simulink model "baseline_super"  (R2021a)
settings: Solver=FixedStepAuto  StartTime=0.0  StopTime=50  FixedStep=framePeriod_s  RelTol=1e-3
undefined symbols (not defined in the file or in its folder): Aircraft, Earth, framePeriod_s, WGS84
libraries: pid_lib x32, simulink x29, aerolibtransform2 x3, simulink_extras x2, aerolibguid x1
(part 3 of 4)

== system baseline_super/LAND CONTROLLER/Horizontal speed controller/Subsystem ==
  vb_x cmd : Inport
  vb_x : Inport  Port=2
  Constant : Constant  Value=Aircraft.Control.P_v_hor  OutDataTypeStr=single
  Constant1 : Constant  Value=Aircraft.Control.I_v_hor  OutDataTypeStr=single
  Constant2 : Constant  Value=Aircraft.Control.D_v_hor  OutDataTypeStr=single
  Gain : Gain  Gain=-1
  Pitch angle controller : pid_lib/PID Controller  Controller=PID  Form=Parallel  TimeDomain=Discrete-time  UseExternalTs=off  SampleTime=framePeriod_s  IntegratorMethod=Forward Euler  FilterMethod=Forward Euler  ControllerParametersSource=external  P=0.335  I=0.005  D=0  UseFilter=off  N=100  TunerSelectOption=Transfer Function Based (PID Tuner App)  InitialConditionSource=internal  InitialConditionForIntegrator=0  InitialConditionForFilter=0  DifferentiatorICPrevScaledInput=0  ExternalReset=none  TrackingMode=off  Kt=1  LimitOutput=on  SatLimitsSource=internal  UpperSaturationLimit=inf  LowerSaturationLimit=-inf  LinearizeAsGain=off  AntiWindupMode=clamping  Kb=1  POutMin=[]  POutMax=[]  IOutMin=[]  IOutMax=[]  DOutMin=[]  DOutMax=[]  NOutMin=[]  NOutMax=[]  SumOutMin=[]  SumOutMax=[]  SaturationOutMin=[]  SaturationOutMax=[]  PParamMin=[]  PParamMax=[]  IParamMin=[]  IParamMax=[]  DParamMin=[]  DParamMax=[]  NParamMin=[]  NParamMax=[]  KbParamMin=[]  KbParamMax=[]  KtParamMin=[]  KtParamMax=[]  KbOutMin=[]  KbOutMax=[]  KtOutMin=[]  KtOutMax=[]  IntegratorOutMin=[]  IntegratorOutMax=[]  FilterOutMin=[]  FilterOutMax=[]  SumI1OutMin=[]  SumI1OutMax=[]  SumI2OutMin=[]  SumI2OutMax=[]  SumI3OutMin=[]  SumI3OutMax=[]  SumI4OutMin=[]  SumI4OutMax=[]  SumDOutMin=[]  SumDOutMax=[]  DifferentiatorOutMin=[]  DifferentiatorOutMax=[]  FilterDiffOutCoefMin=[]  FilterDiffOutCoefMax=[]  ReciprocalOutMin=[]  ReciprocalOutMax=[]  SumDenOutMin=[]  SumDenOutMax=[]  SumNumOutMin=[]  SumNumOutMax=[]  DivideOutMin=[]  DivideOutMax=[]  UdiffTsProdOutMin=[]  UdiffTsProdOutMax=[]  NTsProdOutMin=[]  NTsProdOutMax=[]  UintegralTsProdOutMin=[]  UintegralTsProdOutMax=[]  UngainTsProdOutMin=[]  UngainTsProdOutMax=[]  IntegratorContinuousStateAttributes=''  IntegratorStateMustResolveToSignalObject=off  IntegratorRTWStateStorageClass=Auto  FilterContinuousStateAttributes=''  FilterStateMustResolveToSignalObject=off  FilterRTWStateStorageClass=Auto  ParallelPVariant=ExternalParameters  IdealPVariant=Disabled  IVariant=ExternalParameters  DVariant=ExternalParameters  IntegratorVariant=Discrete  SatVariant=Enabled  AWVariant=DiscClampingParallel  PCopyVariant=Disabled  TRVariant=Disabled  FdbkBlocksVariant=Forward  IdealPFdbkVariant=Disabled  SatFdbkVariant=Disabled  DerivativeFilterVariant=Differentiator  NVariant=Passthrough  NCopyVariant=Disabled_SignalSpec  FilterICVariant=InternalICsDifferentiator  IntegratorICVariant=InternalICs  ExternalResetVariant=Disabled  TRSumVariant=Passthrough  SumFdbkVariant=Disabled  SumVariant=Sum_PID  TsampFilterVariant=InternalTs  TsampNgainVariant=Passthrough  TsampIntegralVariant=Passthrough  ExternalSaturationOutDataTypeStr=Inherit: Same as second input
  Saturation : Saturate  UpperLimit=Aircraft.Control.pitch_angle_lim  LowerLimit=-Aircraft.Control.pitch_angle_lim  LinearizeAsGain=off
  Sum : Sum  Inputs=|+-
  pitch_cmd_rad : Outport
  wires:
  vb_x/1 -> Sum/2
  Constant1/1 -> Pitch angle controller/3
  Constant2/1 -> Pitch angle controller/4
  Sum/1 -> Pitch angle controller/1
  Constant/1 -> Pitch angle controller/2
  vb_x cmd/1 -> Sum/1
  Saturation/1 -> Gain/1
  Pitch angle controller/1 -> Saturation/1
  Gain/1 -> pitch_cmd_rad/1

== system baseline_super/LAND CONTROLLER/Horizontal speed controller/Subsystem1 ==
  vb_y cmd : Inport
  vb_y : Inport  Port=2
  Constant : Constant  Value=Aircraft.Control.P_v_hor  OutDataTypeStr=single
  Constant1 : Constant  Value=Aircraft.Control.I_v_hor  OutDataTypeStr=single
  Constant2 : Constant  Value=Aircraft.Control.D_v_hor  OutDataTypeStr=single
  Roll angle controller : pid_lib/PID Controller  Controller=PID  Form=Parallel  TimeDomain=Discrete-time  UseExternalTs=off  SampleTime=framePeriod_s  IntegratorMethod=Forward Euler  FilterMethod=Forward Euler  ControllerParametersSource=external  P=0.335  I=0.005  D=0  UseFilter=off  N=100  TunerSelectOption=Transfer Function Based (PID Tuner App)  InitialConditionSource=internal  InitialConditionForIntegrator=0  InitialConditionForFilter=0  DifferentiatorICPrevScaledInput=0  ExternalReset=none  TrackingMode=off  Kt=1  LimitOutput=on  SatLimitsSource=internal  UpperSaturationLimit=inf  LowerSaturationLimit=-inf  LinearizeAsGain=off  AntiWindupMode=clamping  Kb=1  POutMin=[]  POutMax=[]  IOutMin=[]  IOutMax=[]  DOutMin=[]  DOutMax=[]  NOutMin=[]  NOutMax=[]  SumOutMin=[]  SumOutMax=[]  SaturationOutMin=[]  SaturationOutMax=[]  PParamMin=[]  PParamMax=[]  IParamMin=[]  IParamMax=[]  DParamMin=[]  DParamMax=[]  NParamMin=[]  NParamMax=[]  KbParamMin=[]  KbParamMax=[]  KtParamMin=[]  KtParamMax=[]  KbOutMin=[]  KbOutMax=[]  KtOutMin=[]  KtOutMax=[]  IntegratorOutMin=[]  IntegratorOutMax=[]  FilterOutMin=[]  FilterOutMax=[]  SumI1OutMin=[]  SumI1OutMax=[]  SumI2OutMin=[]  SumI2OutMax=[]  SumI3OutMin=[]  SumI3OutMax=[]  SumI4OutMin=[]  SumI4OutMax=[]  SumDOutMin=[]  SumDOutMax=[]  DifferentiatorOutMin=[]  DifferentiatorOutMax=[]  FilterDiffOutCoefMin=[]  FilterDiffOutCoefMax=[]  ReciprocalOutMin=[]  ReciprocalOutMax=[]  SumDenOutMin=[]  SumDenOutMax=[]  SumNumOutMin=[]  SumNumOutMax=[]  DivideOutMin=[]  DivideOutMax=[]  UdiffTsProdOutMin=[]  UdiffTsProdOutMax=[]  NTsProdOutMin=[]  NTsProdOutMax=[]  UintegralTsProdOutMin=[]  UintegralTsProdOutMax=[]  UngainTsProdOutMin=[]  UngainTsProdOutMax=[]  IntegratorContinuousStateAttributes=''  IntegratorStateMustResolveToSignalObject=off  IntegratorRTWStateStorageClass=Auto  FilterContinuousStateAttributes=''  FilterStateMustResolveToSignalObject=off  FilterRTWStateStorageClass=Auto  ParallelPVariant=ExternalParameters  IdealPVariant=Disabled  IVariant=ExternalParameters  DVariant=ExternalParameters  IntegratorVariant=Discrete  SatVariant=Enabled  AWVariant=DiscClampingParallel  PCopyVariant=Disabled  TRVariant=Disabled  FdbkBlocksVariant=Forward  IdealPFdbkVariant=Disabled  SatFdbkVariant=Disabled  DerivativeFilterVariant=Differentiator  NVariant=Passthrough  NCopyVariant=Disabled_SignalSpec  FilterICVariant=InternalICsDifferentiator  IntegratorICVariant=InternalICs  ExternalResetVariant=Disabled  TRSumVariant=Passthrough  SumFdbkVariant=Disabled  SumVariant=Sum_PID  TsampFilterVariant=InternalTs  TsampNgainVariant=Passthrough  TsampIntegralVariant=Passthrough  ExternalSaturationOutDataTypeStr=Inherit: Same as second input
  Saturation : Saturate  UpperLimit=Aircraft.Control.pitch_angle_lim  LowerLimit=-Aircraft.Control.pitch_angle_lim  LinearizeAsGain=off
  Sum : Sum  Inputs=|+-
  roll_cmd_rad : Outport
  wires:
  vb_y/1 -> Sum/2
  Constant1/1 -> Roll angle controller/3
  Constant2/1 -> Roll angle controller/4
  Sum/1 -> Roll angle controller/1
  Constant/1 -> Roll angle controller/2
  vb_y cmd/1 -> Sum/1
  Saturation/1 -> roll_cmd_rad/1
  Roll angle controller/1 -> Saturation/1

== system baseline_super/LAND CONTROLLER/auto_disarm/disarm motor ==
  Enable : EnablePort  StatesWhenEnabling=reset
  Compare To Constant2 : simulink/Logic and Bit Operations/Compare To Constant  relop=>  const=10  OutDataTypeStr=boolean
  Constant : Constant  Value=framePeriod_s
  Sum : Sum  Inputs=|++
  Trigger RTL : Subsystem
  Unit Delay : UnitDelay  SampleTime=-1  HasFrameUpgradeWarning=on
  wires:
  Compare To Constant2/1 -> Trigger RTL/Enable
  Sum/1 -> Compare To Constant2/1, Unit Delay/1
  Unit Delay/1 -> Sum/2
  Constant/1 -> Sum/1

== system baseline_super/POS_HOLD CONTROLLER/Horizontal speed controller/2D rotation from NED_xy to body_xy ==
  <heading_rad> : Inport
  Cos : Trigonometry  Operator=cos  OutputSignalType=real
  Gain : Gain  Gain=-1
  Mux : Mux
  Reshape : Reshape  OutputDimensionality=Customize  OutputDimensions=[2,2]
  Sin : Trigonometry  OutputSignalType=real
  2D_rot : Outport
  wires:
  <heading_rad>/1 -> Sin/1, Cos/1
  Mux/1 -> Reshape/1
  Sin/1 -> Mux/3, Gain/1
  Cos/1 -> Mux/1, Mux/4
  Reshape/1 -> 2D_rot/1
  Gain/1 -> Mux/2

== system baseline_super/POS_HOLD CONTROLLER/Horizontal speed controller/Pitch Controller ==
  pitch_cmd_rad : Inport
  pitch_rad : Inport  Port=2
  D_pitch_angle : Constant  Value=Aircraft.Control.I_pitch_angle  OutDataTypeStr=single
  I_pitch_angle : Constant  Value=Aircraft.Control.D_pitch_angle  OutDataTypeStr=single
  P_pitch_angle : Constant  Value=Aircraft.Control.P_pitch_angle  OutDataTypeStr=single
  Pitch angle controller : pid_lib/PID Controller  Controller=PID  Form=Parallel  TimeDomain=Discrete-time  UseExternalTs=off  SampleTime=framePeriod_s  IntegratorMethod=Forward Euler  FilterMethod=Forward Euler  ControllerParametersSource=external  P=0.335  I=0.005  D=0  UseFilter=off  N=100  TunerSelectOption=Transfer Function Based (PID Tuner App)  InitialConditionSource=internal  InitialConditionForIntegrator=0  InitialConditionForFilter=0  DifferentiatorICPrevScaledInput=0  ExternalReset=none  TrackingMode=off  Kt=1  LimitOutput=on  SatLimitsSource=internal  UpperSaturationLimit=inf  LowerSaturationLimit=-inf  LinearizeAsGain=off  AntiWindupMode=clamping  Kb=1  POutMin=[]  POutMax=[]  IOutMin=[]  IOutMax=[]  DOutMin=[]  DOutMax=[]  NOutMin=[]  NOutMax=[]  SumOutMin=[]  SumOutMax=[]  SaturationOutMin=[]  SaturationOutMax=[]  PParamMin=[]  PParamMax=[]  IParamMin=[]  IParamMax=[]  DParamMin=[]  DParamMax=[]  NParamMin=[]  NParamMax=[]  KbParamMin=[]  KbParamMax=[]  KtParamMin=[]  KtParamMax=[]  KbOutMin=[]  KbOutMax=[]  KtOutMin=[]  KtOutMax=[]  IntegratorOutMin=[]  IntegratorOutMax=[]  FilterOutMin=[]  FilterOutMax=[]  SumI1OutMin=[]  SumI1OutMax=[]  SumI2OutMin=[]  SumI2OutMax=[]  SumI3OutMin=[]  SumI3OutMax=[]  SumI4OutMin=[]  SumI4OutMax=[]  SumDOutMin=[]  SumDOutMax=[]  DifferentiatorOutMin=[]  DifferentiatorOutMax=[]  FilterDiffOutCoefMin=[]  FilterDiffOutCoefMax=[]  ReciprocalOutMin=[]  ReciprocalOutMax=[]  SumDenOutMin=[]  SumDenOutMax=[]  SumNumOutMin=[]  SumNumOutMax=[]  DivideOutMin=[]  DivideOutMax=[]  UdiffTsProdOutMin=[]  UdiffTsProdOutMax=[]  NTsProdOutMin=[]  NTsProdOutMax=[]  UintegralTsProdOutMin=[]  UintegralTsProdOutMax=[]  UngainTsProdOutMin=[]  UngainTsProdOutMax=[]  IntegratorContinuousStateAttributes=''  IntegratorStateMustResolveToSignalObject=off  IntegratorRTWStateStorageClass=Auto  FilterContinuousStateAttributes=''  FilterStateMustResolveToSignalObject=off  FilterRTWStateStorageClass=Auto  ParallelPVariant=ExternalParameters  IdealPVariant=Disabled  IVariant=ExternalParameters  DVariant=ExternalParameters  IntegratorVariant=Discrete  SatVariant=Enabled  AWVariant=DiscClampingParallel  PCopyVariant=Disabled  TRVariant=Disabled  FdbkBlocksVariant=Forward  IdealPFdbkVariant=Disabled  SatFdbkVariant=Disabled  DerivativeFilterVariant=Differentiator  NVariant=Passthrough  NCopyVariant=Disabled_SignalSpec  FilterICVariant=InternalICsDifferentiator  IntegratorICVariant=InternalICs  ExternalResetVariant=Disabled  TRSumVariant=Passthrough  SumFdbkVariant=Disabled  SumVariant=Sum_PID  TsampFilterVariant=InternalTs  TsampNgainVariant=Passthrough  TsampIntegralVariant=Passthrough  ExternalSaturationOutDataTypeStr=Inherit: Same as second input
  Saturation : Saturate  UpperLimit=Aircraft.Control.pitch_rate_max  LowerLimit=-Aircraft.Control.pitch_rate_max
  Sum2 : Sum  Inputs=|+-
  pitch_cc : Outport
  wires:
  Sum2/1 -> Pitch angle controller/1  "pitch error"
  P_pitch_angle/1 -> Pitch angle controller/2
  I_pitch_angle/1 -> Pitch angle controller/3
  pitch_cmd_rad/1 -> Sum2/1  "pitch angle cmd"
  D_pitch_angle/1 -> Pitch angle controller/4
  Pitch angle controller/1 -> Saturation/1
  pitch_rad/1 -> Sum2/2
  Saturation/1 -> pitch_cc/1

== system baseline_super/POS_HOLD CONTROLLER/Horizontal speed controller/Roll Controller ==
  roll_cmd_rad : Inport
  roll_rad : Inport  Port=2
  D_roll_angle : Constant  Value=Aircraft.Control.D_roll_angle  OutDataTypeStr=single
  I_roll_angle : Constant  Value=Aircraft.Control.I_roll_angle  OutDataTypeStr=single
  PID Controller1 : pid_lib/PID Controller  Controller=PID  Form=Parallel  TimeDomain=Discrete-time  UseExternalTs=off  SampleTime=framePeriod_s  IntegratorMethod=Forward Euler  FilterMethod=Forward Euler  ControllerParametersSource=external  P=0.335  I=0.005  D=0  UseFilter=off  N=100  TunerSelectOption=Transfer Function Based (PID Tuner App)  InitialConditionSource=internal  InitialConditionForIntegrator=0  InitialConditionForFilter=0  DifferentiatorICPrevScaledInput=0  ExternalReset=none  TrackingMode=off  Kt=1  LimitOutput=on  SatLimitsSource=internal  UpperSaturationLimit=inf  LowerSaturationLimit=-inf  LinearizeAsGain=off  AntiWindupMode=clamping  Kb=1  POutMin=[]  POutMax=[]  IOutMin=[]  IOutMax=[]  DOutMin=[]  DOutMax=[]  NOutMin=[]  NOutMax=[]  SumOutMin=[]  SumOutMax=[]  SaturationOutMin=[]  SaturationOutMax=[]  PParamMin=[]  PParamMax=[]  IParamMin=[]  IParamMax=[]  DParamMin=[]  DParamMax=[]  NParamMin=[]  NParamMax=[]  KbParamMin=[]  KbParamMax=[]  KtParamMin=[]  KtParamMax=[]  KbOutMin=[]  KbOutMax=[]  KtOutMin=[]  KtOutMax=[]  IntegratorOutMin=[]  IntegratorOutMax=[]  FilterOutMin=[]  FilterOutMax=[]  SumI1OutMin=[]  SumI1OutMax=[]  SumI2OutMin=[]  SumI2OutMax=[]  SumI3OutMin=[]  SumI3OutMax=[]  SumI4OutMin=[]  SumI4OutMax=[]  SumDOutMin=[]  SumDOutMax=[]  DifferentiatorOutMin=[]  DifferentiatorOutMax=[]  FilterDiffOutCoefMin=[]  FilterDiffOutCoefMax=[]  ReciprocalOutMin=[]  ReciprocalOutMax=[]  SumDenOutMin=[]  SumDenOutMax=[]  SumNumOutMin=[]  SumNumOutMax=[]  DivideOutMin=[]  DivideOutMax=[]  UdiffTsProdOutMin=[]  UdiffTsProdOutMax=[]  NTsProdOutMin=[]  NTsProdOutMax=[]  UintegralTsProdOutMin=[]  UintegralTsProdOutMax=[]  UngainTsProdOutMin=[]  UngainTsProdOutMax=[]  IntegratorContinuousStateAttributes=''  IntegratorStateMustResolveToSignalObject=off  IntegratorRTWStateStorageClass=Auto  FilterContinuousStateAttributes=''  FilterStateMustResolveToSignalObject=off  FilterRTWStateStorageClass=Auto  ParallelPVariant=ExternalParameters  IdealPVariant=Disabled  IVariant=ExternalParameters  DVariant=ExternalParameters  IntegratorVariant=Discrete  SatVariant=Enabled  AWVariant=DiscClampingParallel  PCopyVariant=Disabled  TRVariant=Disabled  FdbkBlocksVariant=Forward  IdealPFdbkVariant=Disabled  SatFdbkVariant=Disabled  DerivativeFilterVariant=Differentiator  NVariant=Passthrough  NCopyVariant=Disabled_SignalSpec  FilterICVariant=InternalICsDifferentiator  IntegratorICVariant=InternalICs  ExternalResetVariant=Disabled  TRSumVariant=Passthrough  SumFdbkVariant=Disabled  SumVariant=Sum_PID  TsampFilterVariant=InternalTs  TsampNgainVariant=Passthrough  TsampIntegralVariant=Passthrough  ExternalSaturationOutDataTypeStr=Inherit: Same as second input
  P_roll_angle : Constant  Value=Aircraft.Control.P_roll_angle  OutDataTypeStr=single
  Saturation : Saturate  UpperLimit=Aircraft.Control.roll_rate_max  LowerLimit=-Aircraft.Control.roll_rate_max
  Sum : Sum  Inputs=|+-
  roll_cc : Outport
  wires:
  PID Controller1/1 -> Saturation/1  "Roll_cmd"
  roll_cmd_rad/1 -> Sum/1  "roll_angle_command"
  Sum/1 -> PID Controller1/1  "roll_angle_error"
  P_roll_angle/1 -> PID Controller1/2
  I_roll_angle/1 -> PID Controller1/3
  D_roll_angle/1 -> PID Controller1/4
  roll_rad/1 -> Sum/2
  Saturation/1 -> roll_cc/1

== system baseline_super/POS_HOLD CONTROLLER/Horizontal speed controller/Subsystem ==
  vb_x cmd : Inport
  vb_x : Inport  Port=2
  Constant : Constant  Value=Aircraft.Control.P_v_hor  OutDataTypeStr=single
  Constant1 : Constant  Value=Aircraft.Control.I_v_hor  OutDataTypeStr=single
  Constant2 : Constant  Value=Aircraft.Control.D_v_hor  OutDataTypeStr=single
  Gain : Gain  Gain=-1
  Pitch angle controller : pid_lib/PID Controller  Controller=PID  Form=Parallel  TimeDomain=Discrete-time  UseExternalTs=off  SampleTime=framePeriod_s  IntegratorMethod=Forward Euler  FilterMethod=Forward Euler  ControllerParametersSource=external  P=0.335  I=0.005  D=0  UseFilter=off  N=100  TunerSelectOption=Transfer Function Based (PID Tuner App)  InitialConditionSource=internal  InitialConditionForIntegrator=0  InitialConditionForFilter=0  DifferentiatorICPrevScaledInput=0  ExternalReset=none  TrackingMode=off  Kt=1  LimitOutput=on  SatLimitsSource=internal  UpperSaturationLimit=inf  LowerSaturationLimit=-inf  LinearizeAsGain=off  AntiWindupMode=clamping  Kb=1  POutMin=[]  POutMax=[]  IOutMin=[]  IOutMax=[]  DOutMin=[]  DOutMax=[]  NOutMin=[]  NOutMax=[]  SumOutMin=[]  SumOutMax=[]  SaturationOutMin=[]  SaturationOutMax=[]  PParamMin=[]  PParamMax=[]  IParamMin=[]  IParamMax=[]  DParamMin=[]  DParamMax=[]  NParamMin=[]  NParamMax=[]  KbParamMin=[]  KbParamMax=[]  KtParamMin=[]  KtParamMax=[]  KbOutMin=[]  KbOutMax=[]  KtOutMin=[]  KtOutMax=[]  IntegratorOutMin=[]  IntegratorOutMax=[]  FilterOutMin=[]  FilterOutMax=[]  SumI1OutMin=[]  SumI1OutMax=[]  SumI2OutMin=[]  SumI2OutMax=[]  SumI3OutMin=[]  SumI3OutMax=[]  SumI4OutMin=[]  SumI4OutMax=[]  SumDOutMin=[]  SumDOutMax=[]  DifferentiatorOutMin=[]  DifferentiatorOutMax=[]  FilterDiffOutCoefMin=[]  FilterDiffOutCoefMax=[]  ReciprocalOutMin=[]  ReciprocalOutMax=[]  SumDenOutMin=[]  SumDenOutMax=[]  SumNumOutMin=[]  SumNumOutMax=[]  DivideOutMin=[]  DivideOutMax=[]  UdiffTsProdOutMin=[]  UdiffTsProdOutMax=[]  NTsProdOutMin=[]  NTsProdOutMax=[]  UintegralTsProdOutMin=[]  UintegralTsProdOutMax=[]  UngainTsProdOutMin=[]  UngainTsProdOutMax=[]  IntegratorContinuousStateAttributes=''  IntegratorStateMustResolveToSignalObject=off  IntegratorRTWStateStorageClass=Auto  FilterContinuousStateAttributes=''  FilterStateMustResolveToSignalObject=off  FilterRTWStateStorageClass=Auto  ParallelPVariant=ExternalParameters  IdealPVariant=Disabled  IVariant=ExternalParameters  DVariant=ExternalParameters  IntegratorVariant=Discrete  SatVariant=Enabled  AWVariant=DiscClampingParallel  PCopyVariant=Disabled  TRVariant=Disabled  FdbkBlocksVariant=Forward  IdealPFdbkVariant=Disabled  SatFdbkVariant=Disabled  DerivativeFilterVariant=Differentiator  NVariant=Passthrough  NCopyVariant=Disabled_SignalSpec  FilterICVariant=InternalICsDifferentiator  IntegratorICVariant=InternalICs  ExternalResetVariant=Disabled  TRSumVariant=Passthrough  SumFdbkVariant=Disabled  SumVariant=Sum_PID  TsampFilterVariant=InternalTs  TsampNgainVariant=Passthrough  TsampIntegralVariant=Passthrough  ExternalSaturationOutDataTypeStr=Inherit: Same as second input
  Saturation : Saturate  UpperLimit=Aircraft.Control.pitch_angle_lim  LowerLimit=-Aircraft.Control.pitch_angle_lim  LinearizeAsGain=off
  Sum : Sum  Inputs=|+-
  pitch_cmd_rad : Outport
  wires:
  vb_x/1 -> Sum/2
  Constant1/1 -> Pitch angle controller/3
  Constant2/1 -> Pitch angle controller/4
  Sum/1 -> Pitch angle controller/1
  Constant/1 -> Pitch angle controller/2
  vb_x cmd/1 -> Sum/1
  Saturation/1 -> Gain/1
  Pitch angle controller/1 -> Saturation/1
  Gain/1 -> pitch_cmd_rad/1

== system baseline_super/POS_HOLD CONTROLLER/Horizontal speed controller/Subsystem1 ==
  vb_y cmd : Inport
  vb_y : Inport  Port=2
  Constant : Constant  Value=Aircraft.Control.P_v_hor  OutDataTypeStr=single
  Constant1 : Constant  Value=Aircraft.Control.I_v_hor  OutDataTypeStr=single
  Constant2 : Constant  Value=Aircraft.Control.D_v_hor  OutDataTypeStr=single
  Roll angle controller : pid_lib/PID Controller  Controller=PID  Form=Parallel  TimeDomain=Discrete-time  UseExternalTs=off  SampleTime=framePeriod_s  IntegratorMethod=Forward Euler  FilterMethod=Forward Euler  ControllerParametersSource=external  P=0.335  I=0.005  D=0  UseFilter=off  N=100  TunerSelectOption=Transfer Function Based (PID Tuner App)  InitialConditionSource=internal  InitialConditionForIntegrator=0  InitialConditionForFilter=0  DifferentiatorICPrevScaledInput=0  ExternalReset=none  TrackingMode=off  Kt=1  LimitOutput=on  SatLimitsSource=internal  UpperSaturationLimit=inf  LowerSaturationLimit=-inf  LinearizeAsGain=off  AntiWindupMode=clamping  Kb=1  POutMin=[]  POutMax=[]  IOutMin=[]  IOutMax=[]  DOutMin=[]  DOutMax=[]  NOutMin=[]  NOutMax=[]  SumOutMin=[]  SumOutMax=[]  SaturationOutMin=[]  SaturationOutMax=[]  PParamMin=[]  PParamMax=[]  IParamMin=[]  IParamMax=[]  DParamMin=[]  DParamMax=[]  NParamMin=[]  NParamMax=[]  KbParamMin=[]  KbParamMax=[]  KtParamMin=[]  KtParamMax=[]  KbOutMin=[]  KbOutMax=[]  KtOutMin=[]  KtOutMax=[]  IntegratorOutMin=[]  IntegratorOutMax=[]  FilterOutMin=[]  FilterOutMax=[]  SumI1OutMin=[]  SumI1OutMax=[]  SumI2OutMin=[]  SumI2OutMax=[]  SumI3OutMin=[]  SumI3OutMax=[]  SumI4OutMin=[]  SumI4OutMax=[]  SumDOutMin=[]  SumDOutMax=[]  DifferentiatorOutMin=[]  DifferentiatorOutMax=[]  FilterDiffOutCoefMin=[]  FilterDiffOutCoefMax=[]  ReciprocalOutMin=[]  ReciprocalOutMax=[]  SumDenOutMin=[]  SumDenOutMax=[]  SumNumOutMin=[]  SumNumOutMax=[]  DivideOutMin=[]  DivideOutMax=[]  UdiffTsProdOutMin=[]  UdiffTsProdOutMax=[]  NTsProdOutMin=[]  NTsProdOutMax=[]  UintegralTsProdOutMin=[]  UintegralTsProdOutMax=[]  UngainTsProdOutMin=[]  UngainTsProdOutMax=[]  IntegratorContinuousStateAttributes=''  IntegratorStateMustResolveToSignalObject=off  IntegratorRTWStateStorageClass=Auto  FilterContinuousStateAttributes=''  FilterStateMustResolveToSignalObject=off  FilterRTWStateStorageClass=Auto  ParallelPVariant=ExternalParameters  IdealPVariant=Disabled  IVariant=ExternalParameters  DVariant=ExternalParameters  IntegratorVariant=Discrete  SatVariant=Enabled  AWVariant=DiscClampingParallel  PCopyVariant=Disabled  TRVariant=Disabled  FdbkBlocksVariant=Forward  IdealPFdbkVariant=Disabled  SatFdbkVariant=Disabled  DerivativeFilterVariant=Differentiator  NVariant=Passthrough  NCopyVariant=Disabled_SignalSpec  FilterICVariant=InternalICsDifferentiator  IntegratorICVariant=InternalICs  ExternalResetVariant=Disabled  TRSumVariant=Passthrough  SumFdbkVariant=Disabled  SumVariant=Sum_PID  TsampFilterVariant=InternalTs  TsampNgainVariant=Passthrough  TsampIntegralVariant=Passthrough  ExternalSaturationOutDataTypeStr=Inherit: Same as second input
  Saturation : Saturate  UpperLimit=Aircraft.Control.pitch_angle_lim  LowerLimit=-Aircraft.Control.pitch_angle_lim  LinearizeAsGain=off
  Sum : Sum  Inputs=|+-
  roll_cmd_rad : Outport
  wires:
  vb_y/1 -> Sum/2
  Constant1/1 -> Roll angle controller/3
  Constant2/1 -> Roll angle controller/4
  Sum/1 -> Roll angle controller/1
  Constant/1 -> Roll angle controller/2
  Saturation/1 -> roll_cmd_rad/1
  Roll angle controller/1 -> Saturation/1
  vb_y cmd/1 -> Sum/1

== system baseline_super/POS_HOLD CONTROLLER/Vertical speed controller/Throttle Mapper ==
  Throttle : Inport
  Compare To Constant : simulink/Logic and Bit Operations/Compare To Constant  relop=<  const=0  OutDataTypeStr=boolean
  Compare To Constant1 : simulink/Logic and Bit Operations/Compare To Constant  relop=>=  const=0  OutDataTypeStr=boolean
  Constant : Constant  Value=Aircraft.Control.v_z_down_max  OutDataTypeStr=single
  Constant1 : Constant  Value=Aircraft.Control.v_z_up_max  OutDataTypeStr=single
  Double : Constant  Value=2  OutDataTypeStr=single
  Normalize at Zero : Constant  Value=0.5  OutDataTypeStr=single
  Product : Product  Inputs=3
  Product1 : Product  Inputs=3
  Sum : Sum  Inputs=|+-
  Sum1 : Sum
  v_z_cmd (-1 to 1) : Product
  Relative Velocity : Outport
  wires:
  Throttle/1 -> Sum/1
  Normalize at Zero/1 -> Sum/2
  Double/1 -> v_z_cmd (-1 to 1)/2
  Sum/1 -> v_z_cmd (-1 to 1)/1
  Sum1/1 -> Relative Velocity/1
  v_z_cmd (-1 to 1)/1 -> Product1/2, Compare To Constant1/1, Compare To Constant/1, Product/3
  Constant1/1 -> Product1/3
  Compare To Constant1/1 -> Product1/1
  Product/1 -> Sum1/1
  Product1/1 -> Sum1/2
  Constant/1 -> Product/1
  Compare To Constant/1 -> Product/2

== system baseline_super/RTL CONTROLLER/Horizontal_position_controller/convert to ve_cmd ==
  speed_cmd_mps : Inport
  bearing_to_target_rad : Inport  Port=2
  Cos : Trigonometry  Operator=cos
  Product : Product
  Product1 : Product
  Sin : Trigonometry
  ve_x_cmd : Outport
  ve_y_cmd : Outport  Port=2
  wires:
  Product/1 -> ve_x_cmd/1
  speed_cmd_mps/1 -> Product/1, Product1/1
  bearing_to_target_rad/1 -> Cos/1, Sin/1
  Cos/1 -> Product/2
  Sin/1 -> Product1/2
  Product1/1 -> ve_y_cmd/1

== system baseline_super/RTL CONTROLLER/Horizontal_position_controller/inertial_to_body conversion ==
  ve_xy : Inport
  heading_rad : Inport  Port=2
  2D rotation from NED_xy to body_xy : Subsystem
  Demux : Demux  Outputs=2
  Product : Product  Multiplication=Matrix(*)
  vb_x : Outport
  vb_y : Outport  Port=2
  wires:
  Demux/1 -> vb_x/1  "vb_x"
  Product/1 -> Demux/1  "vb_xy"
  heading_rad/1 -> 2D rotation from NED_xy to body_xy/1(<heading_rad>)
  ve_xy/1 -> Product/2
  2D rotation from NED_xy to body_xy/1(2D_rot) -> Product/1
  Demux/2 -> vb_y/1  "vb_y"

== system baseline_super/RTL CONTROLLER/heading_controller/yaw_rate_controller ==
  yaw_rate_cmd_radps : Inport
  gyro_z_radps : Inport  Port=2
  D_yaw_rate : Constant  Value=Aircraft.Control.D_yaw_rate  OutDataTypeStr=single
  I_yaw_rate : Constant  Value=Aircraft.Control.I_yaw_rate  OutDataTypeStr=single
  PID Controller1 : pid_lib/PID Controller  Controller=PID  Form=Parallel  TimeDomain=Discrete-time  UseExternalTs=off  SampleTime=framePeriod_s  IntegratorMethod=Forward Euler  FilterMethod=Forward Euler  ControllerParametersSource=external  P=1.85  I=0.01  D=0  UseFilter=off  N=100  TunerSelectOption=Transfer Function Based (PID Tuner App)  InitialConditionSource=internal  InitialConditionForIntegrator=0  InitialConditionForFilter=0  DifferentiatorICPrevScaledInput=0  ExternalReset=none  TrackingMode=off  Kt=1  LimitOutput=on  SatLimitsSource=internal  UpperSaturationLimit=inf  LowerSaturationLimit=-inf  LinearizeAsGain=on  AntiWindupMode=clamping  Kb=1  POutMin=[]  POutMax=[]  IOutMin=[]  IOutMax=[]  DOutMin=[]  DOutMax=[]  NOutMin=[]  NOutMax=[]  SumOutMin=[]  SumOutMax=[]  SaturationOutMin=[]  SaturationOutMax=[]  PParamMin=[]  PParamMax=[]  IParamMin=[]  IParamMax=[]  DParamMin=[]  DParamMax=[]  NParamMin=[]  NParamMax=[]  KbParamMin=[]  KbParamMax=[]  KtParamMin=[]  KtParamMax=[]  KbOutMin=[]  KbOutMax=[]  KtOutMin=[]  KtOutMax=[]  IntegratorOutMin=[]  IntegratorOutMax=[]  FilterOutMin=[]  FilterOutMax=[]  SumI1OutMin=[]  SumI1OutMax=[]  SumI2OutMin=[]  SumI2OutMax=[]  SumI3OutMin=[]  SumI3OutMax=[]  SumI4OutMin=[]  SumI4OutMax=[]  SumDOutMin=[]  SumDOutMax=[]  DifferentiatorOutMin=[]  DifferentiatorOutMax=[]  FilterDiffOutCoefMin=[]  FilterDiffOutCoefMax=[]  ReciprocalOutMin=[]  ReciprocalOutMax=[]  SumDenOutMin=[]  SumDenOutMax=[]  SumNumOutMin=[]  SumNumOutMax=[]  DivideOutMin=[]  DivideOutMax=[]  UdiffTsProdOutMin=[]  UdiffTsProdOutMax=[]  NTsProdOutMin=[]  NTsProdOutMax=[]  UintegralTsProdOutMin=[]  UintegralTsProdOutMax=[]  UngainTsProdOutMin=[]  UngainTsProdOutMax=[]  IntegratorContinuousStateAttributes=''  IntegratorStateMustResolveToSignalObject=off  IntegratorRTWStateStorageClass=Auto  FilterContinuousStateAttributes=''  FilterStateMustResolveToSignalObject=off  FilterRTWStateStorageClass=Auto  ParallelPVariant=ExternalParameters  IdealPVariant=Disabled  IVariant=ExternalParameters  DVariant=ExternalParameters  IntegratorVariant=Discrete  SatVariant=Enabled  AWVariant=DiscClampingParallel  PCopyVariant=Disabled  TRVariant=Disabled  FdbkBlocksVariant=Forward  IdealPFdbkVariant=Disabled  SatFdbkVariant=Disabled  DerivativeFilterVariant=Differentiator  NVariant=Passthrough  NCopyVariant=Disabled_SignalSpec  FilterICVariant=InternalICsDifferentiator  IntegratorICVariant=InternalICs  ExternalResetVariant=Disabled  TRSumVariant=Passthrough  SumFdbkVariant=Disabled  SumVariant=Sum_PID  TsampFilterVariant=InternalTs  TsampNgainVariant=Passthrough  TsampIntegralVariant=Passthrough  ExternalSaturationOutDataTypeStr=Inherit: Same as second input
  P_yaw_rate : Constant  Value=Aircraft.Control.P_yaw_rate  OutDataTypeStr=single
  Sum2 : Sum  Inputs=|+-
  yaw_cmd : Outport
  wires:
  D_yaw_rate/1 -> PID Controller1/4
  I_yaw_rate/1 -> PID Controller1/3
  Sum2/1 -> PID Controller1/1
  P_yaw_rate/1 -> PID Controller1/2
  PID Controller1/1 -> yaw_cmd/1  "yaw_cc"
  yaw_rate_cmd_radps/1 -> Sum2/1
  gyro_z_radps/1 -> Sum2/2

== system baseline_super/RTL CONTROLLER/horizontal_speed_controller/inertial_to_body conversion ==
  <heading_rad> : Inport
  ve_xy : Inport  Port=2
  2D rotation from NED_xy to body_xy : Subsystem
  Demux : Demux  Outputs=2
  Product : Product  Multiplication=Matrix(*)
  vb_y : Outport
  vb_x : Outport  Port=2
  wires:
  Demux/1 -> vb_x/1  "vb_x"
  Product/1 -> Demux/1  "vb_xy"
  <heading_rad>/1 -> 2D rotation from NED_xy to body_xy/1(<heading_rad>)
  ve_xy/1 -> Product/2
  2D rotation from NED_xy to body_xy/1(2D_rot) -> Product/1
  Demux/2 -> vb_y/1  "vb_y"

== system baseline_super/RTL CONTROLLER/horizontal_speed_controller/vb_x_controller ==
  vb_x cmd : Inport
  vb_x : Inport  Port=2
  Constant3 : Constant  Value=Aircraft.Control.P_v_hor  OutDataTypeStr=single
  Constant4 : Constant  Value=Aircraft.Control.I_v_hor  OutDataTypeStr=single
  Constant5 : Constant  Value=Aircraft.Control.D_v_hor  OutDataTypeStr=single
  Gain : Gain  Gain=-1
  Pitch angle controller : pid_lib/PID Controller  Controller=PID  Form=Parallel  TimeDomain=Discrete-time  UseExternalTs=off  SampleTime=framePeriod_s  IntegratorMethod=Forward Euler  FilterMethod=Forward Euler  ControllerParametersSource=external  P=0.335  I=0.005  D=0  UseFilter=off  N=100  TunerSelectOption=Transfer Function Based (PID Tuner App)  InitialConditionSource=internal  InitialConditionForIntegrator=0  InitialConditionForFilter=0  DifferentiatorICPrevScaledInput=0  ExternalReset=none  TrackingMode=off  Kt=1  LimitOutput=on  SatLimitsSource=internal  UpperSaturationLimit=inf  LowerSaturationLimit=-inf  LinearizeAsGain=off  AntiWindupMode=clamping  Kb=1  POutMin=[]  POutMax=[]  IOutMin=[]  IOutMax=[]  DOutMin=[]  DOutMax=[]  NOutMin=[]  NOutMax=[]  SumOutMin=[]  SumOutMax=[]  SaturationOutMin=[]  SaturationOutMax=[]  PParamMin=[]  PParamMax=[]  IParamMin=[]  IParamMax=[]  DParamMin=[]  DParamMax=[]  NParamMin=[]  NParamMax=[]  KbParamMin=[]  KbParamMax=[]  KtParamMin=[]  KtParamMax=[]  KbOutMin=[]  KbOutMax=[]  KtOutMin=[]  KtOutMax=[]  IntegratorOutMin=[]  IntegratorOutMax=[]  FilterOutMin=[]  FilterOutMax=[]  SumI1OutMin=[]  SumI1OutMax=[]  SumI2OutMin=[]  SumI2OutMax=[]  SumI3OutMin=[]  SumI3OutMax=[]  SumI4OutMin=[]  SumI4OutMax=[]  SumDOutMin=[]  SumDOutMax=[]  DifferentiatorOutMin=[]  DifferentiatorOutMax=[]  FilterDiffOutCoefMin=[]  FilterDiffOutCoefMax=[]  ReciprocalOutMin=[]  ReciprocalOutMax=[]  SumDenOutMin=[]  SumDenOutMax=[]  SumNumOutMin=[]  SumNumOutMax=[]  DivideOutMin=[]  DivideOutMax=[]  UdiffTsProdOutMin=[]  UdiffTsProdOutMax=[]  NTsProdOutMin=[]  NTsProdOutMax=[]  UintegralTsProdOutMin=[]  UintegralTsProdOutMax=[]  UngainTsProdOutMin=[]  UngainTsProdOutMax=[]  IntegratorContinuousStateAttributes=''  IntegratorStateMustResolveToSignalObject=off  IntegratorRTWStateStorageClass=Auto  FilterContinuousStateAttributes=''  FilterStateMustResolveToSignalObject=off  FilterRTWStateStorageClass=Auto  ParallelPVariant=ExternalParameters  IdealPVariant=Disabled  IVariant=ExternalParameters  DVariant=ExternalParameters  IntegratorVariant=Discrete  SatVariant=Enabled  AWVariant=DiscClampingParallel  PCopyVariant=Disabled  TRVariant=Disabled  FdbkBlocksVariant=Forward  IdealPFdbkVariant=Disabled  SatFdbkVariant=Disabled  DerivativeFilterVariant=Differentiator  NVariant=Passthrough  NCopyVariant=Disabled_SignalSpec  FilterICVariant=InternalICsDifferentiator  IntegratorICVariant=InternalICs  ExternalResetVariant=Disabled  TRSumVariant=Passthrough  SumFdbkVariant=Disabled  SumVariant=Sum_PID  TsampFilterVariant=InternalTs  TsampNgainVariant=Passthrough  TsampIntegralVariant=Passthrough  ExternalSaturationOutDataTypeStr=Inherit: Same as second input
  Saturation : Saturate  UpperLimit=Aircraft.Control.pitch_angle_lim  LowerLimit=-Aircraft.Control.pitch_angle_lim  LinearizeAsGain=off
  Sum : Sum  Inputs=|+-
  pitch_cmd_rad : Outport
  wires:
  vb_x/1 -> Sum/2
  Constant4/1 -> Pitch angle controller/3
  Constant5/1 -> Pitch angle controller/4
  Sum/1 -> Pitch angle controller/1
  Constant3/1 -> Pitch angle controller/2
  vb_x cmd/1 -> Sum/1
  Saturation/1 -> Gain/1
  Pitch angle controller/1 -> Saturation/1
  Gain/1 -> pitch_cmd_rad/1

== system baseline_super/RTL CONTROLLER/horizontal_speed_controller/vb_y_controller ==
  vb_y cmd : Inport
  vb_y : Inport  Port=2
  Constant : Constant  Value=Aircraft.Control.P_v_hor  OutDataTypeStr=single
  Constant1 : Constant  Value=Aircraft.Control.I_v_hor  OutDataTypeStr=single
  Constant2 : Constant  Value=Aircraft.Control.D_v_hor  OutDataTypeStr=single
  Roll angle controller : pid_lib/PID Controller  Controller=PID  Form=Parallel  TimeDomain=Discrete-time  UseExternalTs=off  SampleTime=framePeriod_s  IntegratorMethod=Forward Euler  FilterMethod=Forward Euler  ControllerParametersSource=external  P=0.335  I=0.005  D=0  UseFilter=off  N=100  TunerSelectOption=Transfer Function Based (PID Tuner App)  InitialConditionSource=internal  InitialConditionForIntegrator=0  InitialConditionForFilter=0  DifferentiatorICPrevScaledInput=0  ExternalReset=none  TrackingMode=off  Kt=1  LimitOutput=on  SatLimitsSource=internal  UpperSaturationLimit=inf  LowerSaturationLimit=-inf  LinearizeAsGain=off  AntiWindupMode=clamping  Kb=1  POutMin=[]  POutMax=[]  IOutMin=[]  IOutMax=[]  DOutMin=[]  DOutMax=[]  NOutMin=[]  NOutMax=[]  SumOutMin=[]  SumOutMax=[]  SaturationOutMin=[]  SaturationOutMax=[]  PParamMin=[]  PParamMax=[]  IParamMin=[]  IParamMax=[]  DParamMin=[]  DParamMax=[]  NParamMin=[]  NParamMax=[]  KbParamMin=[]  KbParamMax=[]  KtParamMin=[]  KtParamMax=[]  KbOutMin=[]  KbOutMax=[]  KtOutMin=[]  KtOutMax=[]  IntegratorOutMin=[]  IntegratorOutMax=[]  FilterOutMin=[]  FilterOutMax=[]  SumI1OutMin=[]  SumI1OutMax=[]  SumI2OutMin=[]  SumI2OutMax=[]  SumI3OutMin=[]  SumI3OutMax=[]  SumI4OutMin=[]  SumI4OutMax=[]  SumDOutMin=[]  SumDOutMax=[]  DifferentiatorOutMin=[]  DifferentiatorOutMax=[]  FilterDiffOutCoefMin=[]  FilterDiffOutCoefMax=[]  ReciprocalOutMin=[]  ReciprocalOutMax=[]  SumDenOutMin=[]  SumDenOutMax=[]  SumNumOutMin=[]  SumNumOutMax=[]  DivideOutMin=[]  DivideOutMax=[]  UdiffTsProdOutMin=[]  UdiffTsProdOutMax=[]  NTsProdOutMin=[]  NTsProdOutMax=[]  UintegralTsProdOutMin=[]  UintegralTsProdOutMax=[]  UngainTsProdOutMin=[]  UngainTsProdOutMax=[]  IntegratorContinuousStateAttributes=''  IntegratorStateMustResolveToSignalObject=off  IntegratorRTWStateStorageClass=Auto  FilterContinuousStateAttributes=''  FilterStateMustResolveToSignalObject=off  FilterRTWStateStorageClass=Auto  ParallelPVariant=ExternalParameters  IdealPVariant=Disabled  IVariant=ExternalParameters  DVariant=ExternalParameters  IntegratorVariant=Discrete  SatVariant=Enabled  AWVariant=DiscClampingParallel  PCopyVariant=Disabled  TRVariant=Disabled  FdbkBlocksVariant=Forward  IdealPFdbkVariant=Disabled  SatFdbkVariant=Disabled  DerivativeFilterVariant=Differentiator  NVariant=Passthrough  NCopyVariant=Disabled_SignalSpec  FilterICVariant=InternalICsDifferentiator  IntegratorICVariant=InternalICs  ExternalResetVariant=Disabled  TRSumVariant=Passthrough  SumFdbkVariant=Disabled  SumVariant=Sum_PID  TsampFilterVariant=InternalTs  TsampNgainVariant=Passthrough  TsampIntegralVariant=Passthrough  ExternalSaturationOutDataTypeStr=Inherit: Same as second input
  Saturation : Saturate  UpperLimit=Aircraft.Control.pitch_angle_lim  LowerLimit=-Aircraft.Control.pitch_angle_lim  LinearizeAsGain=off
  Sum : Sum  Inputs=|+-
  roll_cmd_rad : Outport
  wires:
  vb_y/1 -> Sum/2
  Constant1/1 -> Roll angle controller/3
  Constant2/1 -> Roll angle controller/4
  Sum/1 -> Roll angle controller/1
  Constant/1 -> Roll angle controller/2
  vb_y cmd/1 -> Sum/1
  Saturation/1 -> roll_cmd_rad/1
  Roll angle controller/1 -> Saturation/1

== system baseline_super/RTL CONTROLLER/pitch_roll_angle_controller/Pitch Controller ==
  pitch_cmd_rad : Inport
  pitch_rad : Inport  Port=2
  D_pitch_angle : Constant  Value=Aircraft.Control.I_pitch_angle  OutDataTypeStr=single
  I_pitch_angle : Constant  Value=Aircraft.Control.D_pitch_angle  OutDataTypeStr=single
  P_pitch_angle : Constant  Value=Aircraft.Control.P_pitch_angle  OutDataTypeStr=single
  Pitch angle controller : pid_lib/PID Controller  Controller=PID  Form=Parallel  TimeDomain=Discrete-time  UseExternalTs=off  SampleTime=framePeriod_s  IntegratorMethod=Forward Euler  FilterMethod=Forward Euler  ControllerParametersSource=external  P=0.335  I=0.005  D=0  UseFilter=off  N=100  TunerSelectOption=Transfer Function Based (PID Tuner App)  InitialConditionSource=internal  InitialConditionForIntegrator=0  InitialConditionForFilter=0  DifferentiatorICPrevScaledInput=0  ExternalReset=none  TrackingMode=off  Kt=1  LimitOutput=on  SatLimitsSource=internal  UpperSaturationLimit=inf  LowerSaturationLimit=-inf  LinearizeAsGain=off  AntiWindupMode=clamping  Kb=1  POutMin=[]  POutMax=[]  IOutMin=[]  IOutMax=[]  DOutMin=[]  DOutMax=[]  NOutMin=[]  NOutMax=[]  SumOutMin=[]  SumOutMax=[]  SaturationOutMin=[]  SaturationOutMax=[]  PParamMin=[]  PParamMax=[]  IParamMin=[]  IParamMax=[]  DParamMin=[]  DParamMax=[]  NParamMin=[]  NParamMax=[]  KbParamMin=[]  KbParamMax=[]  KtParamMin=[]  KtParamMax=[]  KbOutMin=[]  KbOutMax=[]  KtOutMin=[]  KtOutMax=[]  IntegratorOutMin=[]  IntegratorOutMax=[]  FilterOutMin=[]  FilterOutMax=[]  SumI1OutMin=[]  SumI1OutMax=[]  SumI2OutMin=[]  SumI2OutMax=[]  SumI3OutMin=[]  SumI3OutMax=[]  SumI4OutMin=[]  SumI4OutMax=[]  SumDOutMin=[]  SumDOutMax=[]  DifferentiatorOutMin=[]  DifferentiatorOutMax=[]  FilterDiffOutCoefMin=[]  FilterDiffOutCoefMax=[]  ReciprocalOutMin=[]  ReciprocalOutMax=[]  SumDenOutMin=[]  SumDenOutMax=[]  SumNumOutMin=[]  SumNumOutMax=[]  DivideOutMin=[]  DivideOutMax=[]  UdiffTsProdOutMin=[]  UdiffTsProdOutMax=[]  NTsProdOutMin=[]  NTsProdOutMax=[]  UintegralTsProdOutMin=[]  UintegralTsProdOutMax=[]  UngainTsProdOutMin=[]  UngainTsProdOutMax=[]  IntegratorContinuousStateAttributes=''  IntegratorStateMustResolveToSignalObject=off  IntegratorRTWStateStorageClass=Auto  FilterContinuousStateAttributes=''  FilterStateMustResolveToSignalObject=off  FilterRTWStateStorageClass=Auto  ParallelPVariant=ExternalParameters  IdealPVariant=Disabled  IVariant=ExternalParameters  DVariant=ExternalParameters  IntegratorVariant=Discrete  SatVariant=Enabled  AWVariant=DiscClampingParallel  PCopyVariant=Disabled  TRVariant=Disabled  FdbkBlocksVariant=Forward  IdealPFdbkVariant=Disabled  SatFdbkVariant=Disabled  DerivativeFilterVariant=Differentiator  NVariant=Passthrough  NCopyVariant=Disabled_SignalSpec  FilterICVariant=InternalICsDifferentiator  IntegratorICVariant=InternalICs  ExternalResetVariant=Disabled  TRSumVariant=Passthrough  SumFdbkVariant=Disabled  SumVariant=Sum_PID  TsampFilterVariant=InternalTs  TsampNgainVariant=Passthrough  TsampIntegralVariant=Passthrough  ExternalSaturationOutDataTypeStr=Inherit: Same as second input
  Saturation : Saturate  UpperLimit=Aircraft.Control.pitch_rate_max  LowerLimit=-Aircraft.Control.pitch_rate_max
  Sum2 : Sum  Inputs=|+-
  pitch_cc : Outport
  wires:
  Sum2/1 -> Pitch angle controller/1  "pitch error"
  P_pitch_angle/1 -> Pitch angle controller/2
  I_pitch_angle/1 -> Pitch angle controller/3
  pitch_cmd_rad/1 -> Sum2/1  "pitch angle cmd"
  D_pitch_angle/1 -> Pitch angle controller/4
  Pitch angle controller/1 -> Saturation/1
  pitch_rad/1 -> Sum2/2
  Saturation/1 -> pitch_cc/1

== system baseline_super/RTL CONTROLLER/pitch_roll_angle_controller/Roll Controller ==
  roll_cmd_rad : Inport
  roll_rad : Inport  Port=2
  D_roll_angle : Constant  Value=Aircraft.Control.D_roll_angle  OutDataTypeStr=single
  I_roll_angle : Constant  Value=Aircraft.Control.I_roll_angle  OutDataTypeStr=single
  PID Controller1 : pid_lib/PID Controller  Controller=PID  Form=Parallel  TimeDomain=Discrete-time  UseExternalTs=off  SampleTime=framePeriod_s  IntegratorMethod=Forward Euler  FilterMethod=Forward Euler  ControllerParametersSource=external  P=0.335  I=0.005  D=0  UseFilter=off  N=100  TunerSelectOption=Transfer Function Based (PID Tuner App)  InitialConditionSource=internal  InitialConditionForIntegrator=0  InitialConditionForFilter=0  DifferentiatorICPrevScaledInput=0  ExternalReset=none  TrackingMode=off  Kt=1  LimitOutput=on  SatLimitsSource=internal  UpperSaturationLimit=inf  LowerSaturationLimit=-inf  LinearizeAsGain=off  AntiWindupMode=clamping  Kb=1  POutMin=[]  POutMax=[]  IOutMin=[]  IOutMax=[]  DOutMin=[]  DOutMax=[]  NOutMin=[]  NOutMax=[]  SumOutMin=[]  SumOutMax=[]  SaturationOutMin=[]  SaturationOutMax=[]  PParamMin=[]  PParamMax=[]  IParamMin=[]  IParamMax=[]  DParamMin=[]  DParamMax=[]  NParamMin=[]  NParamMax=[]  KbParamMin=[]  KbParamMax=[]  KtParamMin=[]  KtParamMax=[]  KbOutMin=[]  KbOutMax=[]  KtOutMin=[]  KtOutMax=[]  IntegratorOutMin=[]  IntegratorOutMax=[]  FilterOutMin=[]  FilterOutMax=[]  SumI1OutMin=[]  SumI1OutMax=[]  SumI2OutMin=[]  SumI2OutMax=[]  SumI3OutMin=[]  SumI3OutMax=[]  SumI4OutMin=[]  SumI4OutMax=[]  SumDOutMin=[]  SumDOutMax=[]  DifferentiatorOutMin=[]  DifferentiatorOutMax=[]  FilterDiffOutCoefMin=[]  FilterDiffOutCoefMax=[]  ReciprocalOutMin=[]  ReciprocalOutMax=[]  SumDenOutMin=[]  SumDenOutMax=[]  SumNumOutMin=[]  SumNumOutMax=[]  DivideOutMin=[]  DivideOutMax=[]  UdiffTsProdOutMin=[]  UdiffTsProdOutMax=[]  NTsProdOutMin=[]  NTsProdOutMax=[]  UintegralTsProdOutMin=[]  UintegralTsProdOutMax=[]  UngainTsProdOutMin=[]  UngainTsProdOutMax=[]  IntegratorContinuousStateAttributes=''  IntegratorStateMustResolveToSignalObject=off  IntegratorRTWStateStorageClass=Auto  FilterContinuousStateAttributes=''  FilterStateMustResolveToSignalObject=off  FilterRTWStateStorageClass=Auto  ParallelPVariant=ExternalParameters  IdealPVariant=Disabled  IVariant=ExternalParameters  DVariant=ExternalParameters  IntegratorVariant=Discrete  SatVariant=Enabled  AWVariant=DiscClampingParallel  PCopyVariant=Disabled  TRVariant=Disabled  FdbkBlocksVariant=Forward  IdealPFdbkVariant=Disabled  SatFdbkVariant=Disabled  DerivativeFilterVariant=Differentiator  NVariant=Passthrough  NCopyVariant=Disabled_SignalSpec  FilterICVariant=InternalICsDifferentiator  IntegratorICVariant=InternalICs  ExternalResetVariant=Disabled  TRSumVariant=Passthrough  SumFdbkVariant=Disabled  SumVariant=Sum_PID  TsampFilterVariant=InternalTs  TsampNgainVariant=Passthrough  TsampIntegralVariant=Passthrough  ExternalSaturationOutDataTypeStr=Inherit: Same as second input
  P_roll_angle : Constant  Value=Aircraft.Control.P_roll_angle  OutDataTypeStr=single
  Saturation : Saturate  UpperLimit=Aircraft.Control.roll_rate_max  LowerLimit=-Aircraft.Control.roll_rate_max
  Sum : Sum  Inputs=|+-
  roll_cc : Outport
  wires:
  PID Controller1/1 -> Saturation/1  "Roll_cmd"
  roll_cmd_rad/1 -> Sum/1  "roll_angle_command"
  Sum/1 -> PID Controller1/1  "roll_angle_error"
  P_roll_angle/1 -> PID Controller1/2
  I_roll_angle/1 -> PID Controller1/3
  D_roll_angle/1 -> PID Controller1/4
  roll_rad/1 -> Sum/2
  Saturation/1 -> roll_cc/1

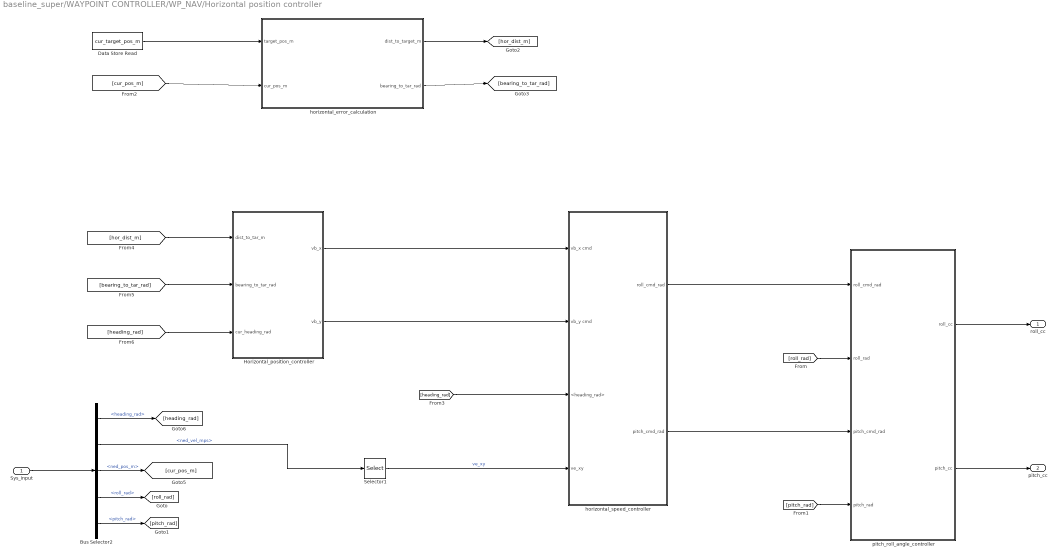
== system baseline_super/WAYPOINT CONTROLLER/WP_NAV/Horizontal position controller ==
  Sys_input : Inport
  Bus Selector2 : BusSelector  OutputSignals=Navigation Filter Data.heading_rad,Navigation Filter Data.ned_vel_mps,Navigation Filter Data.ned_pos_m,Navigation Filter Data.roll_rad,Navigation Filter Data.pitch_rad
  Data Store Read : DataStoreRead  DataStoreName=cur_target_pos_m  IndexOptions=Index vector (dialog)  Indices=1  OutputSizes=1
  Horizontal_position_controller : Subsystem
  Selector1 : Selector  InputPortWidth=3  IndexOptions=Index vector (dialog)  Indices=[1 2]  OutputSizes=1
  "horizontal_error_calculation " : Subsystem
  horizontal_speed_controller : Subsystem
  pitch_roll_angle_controller : Subsystem
  roll_cc : Outport
  pitch_cc : Outport  Port=2
  wires:
  Bus Selector2/4 -> [roll_rad]  "<roll_rad>"
  [pitch_rad] -> pitch_roll_angle_controller/4(pitch_rad)
  Bus Selector2/3 -> [cur_pos_m]  "<ned_pos_m>"
  Bus Selector2/5 -> [pitch_rad]  "<pitch_rad>"
  Bus Selector2/1 -> [heading_rad]  "<heading_rad>"
  Bus Selector2/2 -> Selector1/1  "<ned_vel_mps>"
  [heading_rad] -> horizontal_speed_controller/3(<heading_rad>)
  horizontal_speed_controller/1(roll_cmd_rad) -> pitch_roll_angle_controller/1(roll_cmd_rad)
  [roll_rad] -> pitch_roll_angle_controller/2(roll_rad)
  Selector1/1 -> horizontal_speed_controller/4(ve_xy)  "ve_xy"
  horizontal_speed_controller/2(pitch_cmd_rad) -> pitch_roll_angle_controller/3(pitch_cmd_rad)
  pitch_roll_angle_controller/1(roll_cc) -> roll_cc/1
  pitch_roll_angle_controller/2(pitch_cc) -> pitch_cc/1
  Sys_input/1 -> Bus Selector2/1
  [hor_dist_m] -> Horizontal_position_controller/1(dist_to_tar_m)
  Horizontal_position_controller/1(vb_x) -> horizontal_speed_controller/1(vb_x cmd)
  Horizontal_position_controller/2(vb_y) -> horizontal_speed_controller/2(vb_y cmd)
  [bearing_to_tar_rad] -> Horizontal_position_controller/2(bearing_to_tar_rad)
  [heading_rad] -> Horizontal_position_controller/3(cur_heading_rad)
  Data Store Read/1 -> "horizontal_error_calculation "/1(target_pos_m)
  [cur_pos_m] -> "horizontal_error_calculation "/2(cur_pos_m)
  "horizontal_error_calculation "/1(dist_to_target_m) -> [hor_dist_m]
  "horizontal_error_calculation "/2(bearing_to_tar_rad) -> [bearing_to_tar_rad]

== system baseline_super/WAYPOINT CONTROLLER/WP_NAV/Vertical position controller ==
  Sys_input : Inport
  Bus Selector6 : BusSelector  OutputSignals=Navigation Filter Data.ned_pos_m,Navigation Filter Data.ned_vel_mps
  Data Store Read : DataStoreRead  DataStoreName=cur_target_pos_m  IndexOptions=Index vector (dialog)  Indices=1  OutputSizes=1
  Selector1 : Selector  InputPortWidth=3  IndexOptions=Index vector (dialog)  Indices=3  OutputSizes=1
  select_cur_z : Selector  InputPortWidth=3  IndexOptions=Index vector (dialog)  Indices=3  OutputSizes=1
  select_ned_v_z : Selector  InputPortWidth=3  IndexOptions=Index vector (dialog)  Indices=[3]  OutputSizes=1
  vertical_position_controller : Subsystem
  vertical_speed_controller : Subsystem
  throttle_out : Outport
  wires:
  Sys_input/1 -> Bus Selector6/1
  Bus Selector6/1 -> select_cur_z/1  "<ned_pos_m>"
  Bus Selector6/2 -> select_ned_v_z/1  "<ned_vel_mps>"
  select_ned_v_z/1 -> vertical_speed_controller/2(ve_z_mps)
  vertical_speed_controller/1(throttle) -> throttle_out/1
  Selector1/1 -> vertical_position_controller/1(target_z_m)  "target_z"
  select_cur_z/1 -> vertical_position_controller/2(cur_z_m)
  vertical_position_controller/1(ve_z_cmd) -> vertical_speed_controller/1(ve_z_cmd)
  Data Store Read/1 -> Selector1/1

== system baseline_super/WAYPOINT CONTROLLER/WP_NAV/heading_controller ==
  Sys_input : Inport
  Bus Selector4 : BusSelector  OutputSignals=Navigation Filter Data.heading_rad,Navigation Filter Data.gyro_radps
  Data Store Read1 : DataStoreRead  DataStoreName=cur_target_heading_rad  IndexOptions=Index vector (dialog)  Indices=1  OutputSizes=1
  Selector2 : Selector  InputPortWidth=3  IndexOptions=Index vector (dialog)  Indices=3  OutputSizes=1
  heading_controller : Subsystem
  yaw_rate_controller : Subsystem
  yaw_cc : Outport
  wires:
  Bus Selector4/2 -> Selector2/1  "<gyro_radps>"
  Sys_input/1 -> Bus Selector4/1
  Data Store Read1/1 -> heading_controller/1(heading_cmd_rad)
  Bus Selector4/1 -> heading_controller/2(<heading_rad>)  "<heading_rad>"
  heading_controller/1(yaw_rate_cmd) -> yaw_rate_controller/1(yaw_rate_cmd_radps)
  yaw_rate_controller/1(yaw_cmd) -> yaw_cc/1
  Selector2/1 -> yaw_rate_controller/2(gyro_z_radps)
